simulink model "Flexible_Spacecraft"  (R2019a)
settings: Solver=ode4  StartTime=0.0  StopTime=10  FixedStep=0.005  RelTol=1e-3
libraries: aerolibconvert2 x5
settings Model: Creator=hoomaan  LastModifiedBy=hoomaan
settings DataIOCC: ReturnWorkspaceOutputs=off
settings DebuggingCC: ArithmeticOperatorsInVariantConditions=warning
settings SFSimCC: SimUseLocalCustomCode=off
settings RTWCC: RTWUseLocalCustomCode=off
settings CodeAppCC: StateflowObjectComments=on

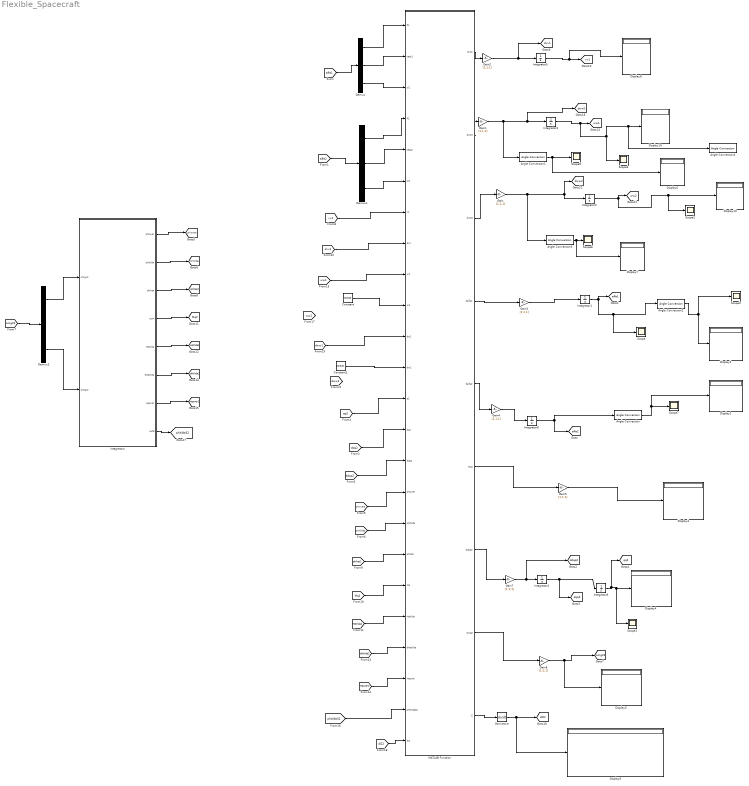
== system Flexible_Spacecraft ==
  Angle Conversion{,1..4} (5 alike) : aerolibconvert2/Angle Conversion  IU=rad  OU=deg
  Constant : Constant  Value=[0;0;0]
  Constant1 : Constant  Value=[0;0;0]
  Demux : Demux  Outputs=3
  Demux1 : Demux  Outputs=3
  Demux2 : Demux  Outputs=3
  Derivative : Derivative
  Display{1..10,13} (11 alike) : Display
  Gain{,1..5,7..8} (8 alike) : Gain  Gain=[1;1;1]
  Integrator{1..6,8} (7 alike) : Integrator  InitialCondition=[0;0;0]
  MATLAB Function : MATLAB Function  TreatAsAtomicUnit=on
  Scope{,1..7} (8 alike) : Scope
  integrators : MATLAB Function  TreatAsAtomicUnit=on
  tag scope: Hqover2=global, Hqtilda2=global, Mq2=global, alfa1=global, alfa2=global, dHtilda2=global, dI22=global, ddqq2=global, dqq2=global, dvv1=global, dww1=global, dww2=global, omg22=global, phihat2=global, phiover2=global, phitilda2=global, phitilda32=global, qq2=global, vv1=global, ww1=global, ww2=global
  wires:
  Angle Conversion/1 -> Scope7/1, Display1/1
  Integrator8/1 -> Angle Conversion/1, [alfa2]
  Integrator1/1 -> [alfa1], Scope/1, Angle Conversion2/1
  [alfa2] -> Demux1/1
  [alfa1] -> Demux/1
  Angle Conversion2/1 -> Scope3/1, Display2/1
  MATLAB Function/1(dv10) -> Gain2/1
  Integrator5/1 -> Display8/1, [vv1]
  MATLAB Function/2(dw10) -> Gain1/1
  MATLAB Function/3(dw20) -> Gain/1
  Integrator2/1 -> [ww2], Scope2/1, Display13/1
  [vv1] -> MATLAB Function/7(v1)
  [ww1] -> MATLAB Function/9(w1)
  [dww1] -> MATLAB Function/11(dw1)
  [dvv1] -> MATLAB Function/8(dv1)
  MATLAB Function/4(dalfa1) -> Gain3/1
  MATLAB Function/5(dalfa2) -> Gain4/1
  Gain/1 -> Angle Conversion3/1, Integrator2/1, [dww2]
  Gain1/1 -> Angle Conversion1/1, Integrator3/1, [dww1]
  Gain2/1 -> Integrator5/1, [dvv1]
  Gain3/1 -> Integrator1/1
  Gain4/1 -> Integrator8/1
  MATLAB Function/6(Mp2) -> Gain5/1
  Gain5/1 -> Display3/1
  Demux1/1 -> MATLAB Function/4(fi2)
  Demux1/2 -> MATLAB Function/5(teta2)
  Demux1/3 -> MATLAB Function/6(si2)
  Demux/1 -> MATLAB Function/1(fi1)
  Demux/2 -> MATLAB Function/2(teta1)
  Demux/3 -> MATLAB Function/3(si1)
  [dqq2] -> MATLAB Function/14(dq2)
  [ddqq2] -> MATLAB Function/15(ddq2)
  MATLAB Function/7(ddq20) -> Gain7/1
  Integrator4/1 -> [dqq2], Integrator6/1
  Integrator6/1 -> Scope1/1, Display4/1, [qq2]
  [qq2] -> MATLAB Function/13(q2)
  Gain7/1 -> [ddqq2], Integrator4/1
  MATLAB Function/8(omg2) -> Gain8/1
  Gain8/1 -> Display5/1, [omg22]
  [omg22] -> Demux2/1
  Demux2/1 -> integrators/1(omgx2)
  Demux2/3 -> integrators/2(omgz2)
  integrators/7(Hqover) -> [Hqover2]
  integrators/6(dHqtilda) -> [dHtilda2]
  integrators/5(Hqtilda) -> [Hqtilda2]
  integrators/4(out4) -> [Mq2]
  integrators/3(phihat) -> [phihat2]
  integrators/2(phitilda) -> [phitilda2]
  integrators/1(phiover) -> [phiover2]
  [phihat2] -> MATLAB Function/18(phihat)
  [phitilda2] -> MATLAB Function/17(phitilda)
  [phiover2] -> MATLAB Function/16(phiover)
  [Mq2] -> MATLAB Function/19(Mq)
  [Hqtilda2] -> MATLAB Function/20(Hqtilda)
  [dHtilda2] -> MATLAB Function/21(dHqtilda)
  [Hqover2] -> MATLAB Function/22(Hqover)
  Angle Conversion1/1 -> Display6/1, Scope5/1
  Angle Conversion3/1 -> Display7/1, Scope6/1
  integrators/8(out8) -> [phitilda32]
  [phitilda32] -> MATLAB Function/23(phitilda32)
  MATLAB Function/9(I2) -> Derivative/1
  Derivative/1 -> Display9/1, [dI22]
  [dI22] -> MATLAB Function/24(dI2)
  Constant/1 -> MATLAB Function/10(w2)
  Constant1/1 -> MATLAB Function/12(dw2)
  Integrator3/1 -> Scope4/1, Angle Conversion4/1, Display10/1, [ww1]

== matlab function Flexible_Spacecraft/integrators ==
  data: omgx2 input; phiover output; omgz2 input; phitilda output; phihat output; out4 output; Hqtilda output; dHqtilda output; Hqover output; out8 output
function [phiover,phitilda,phihat,out4,Hqtilda,dHqtilda,Hqover,out8] = integrators(omgx2,omgz2)
%#codegen

%    This function was generated by the Symbolic Math Toolbox version 7.1.
%    26-Feb-2017 23:02:28

phiover = reshape([0.0,0.0,0.0,0.0,-6.377876326171868,0.0,0.0,0.0,0.0],[3,3]);
if nargout > 1
    phitilda = reshape([0.0,0.0,0.0,0.0,0.0,-1.075141769112719e1,0.0,0.0,0.0],[3,3]);
end
if nargout > 2
    phihat = reshape([0.0,0.0,0.0,0.0,omgx2.*1.075141769112719e1,0.0,0.0,0.0,0.0],[3,3]);
end
if nargout > 3
    out4 = 1.008336895295853;
end
if nargout > 4
    t2 = reshape([0.0,0.0,0.0,0.0,0.0,0.0,0.0,0.0,0.0],[3,3]);
    Hqtilda = t2;
end
if nargout > 5
    dHqtilda = t2;
end
if nargout > 6
    Hqover = reshape([0.0,0.0,0.0,0.0,omgx2.^2.*(-1.008336895295853)-omgz2.^2.*1.008336895295853,0.0,0.0,0.0,0.0],[3,3]);
end
if nargout > 7
    out8 = -1.075141769112719e1;
end

== matlab function Flexible_Spacecraft/MATLAB Function ==
  data: fi1 input; teta1 input; dv10 output; dw10 output; dw20 output; si1 input; fi2 input; teta2 input; si2 input; v1 input; dv1 input; w1 input; w2 input; dw1 input; dw2 input; q2 input; dalfa1 output; dalfa2 output; Mp2 output; dq2 input; ddq20 output; ddq2 input; omg2 output; phiover input; phitilda input; phihat input; Mq input; Hqtilda input; dHqtilda input; Hqover input; phitilda32 input; dI2 input; I2 output
function [dv10,dw10,dw20,dalfa1,dalfa2,Mp2,ddq20,omg2,I2] = fcn(fi1,teta1,si1,fi2,teta2,si2,v1,dv1,w1,w2,dw1,dw2,q2,dq2,ddq2,phiover,phitilda,phihat,Mq,Hqtilda,dHqtilda,Hqover,phitilda32,dI2)

C10=[cos(teta1)*cos(si1) cos(fi1)*sin(si1)+sin(fi1)*sin(teta1)*cos(si1) sin(fi1)*sin(si1)-cos(fi1)*sin(teta1)*cos(si1);-cos(teta1)*sin(si1) cos(fi1)*cos(si1)-sin(fi1)*sin(teta1)*sin(si1) sin(fi1)*cos(si1)+cos(fi1)*sin(teta1)*sin(si1);sin(teta1) -sin(fi1)*cos(teta1) cos(fi1)*cos(teta1)];
C21=[1 0 0;0 1 0;0 0 1];
C12=C21';

D1=[cos(teta1)*cos(si1) sin(si1) 0;-cos(teta1)*sin(si1) cos(si1) 0;sin(teta1) 0 1];
D2=D1;

ro1=2740;
A1=1*1;
ro2=2740;
A2=1*0.01;
h2=0.01;

m1=2740;
m2=205.5;


r1=[1;0;0];
r2=[7.5;0;0];

s1=m1*[0.5;0;0];
s2=m2*[7.5/2;0;0];
j2=s2+(phiover*q2);

I1=[456.6666666667 0 0;0  1.141666666666667e+03 0;0 0  1.141666666666667e+03];
I2=[1.712671250000000e+01+(q2(2,1)*Mq*q2(2,1)) -phitilda32*q2(2,1) 0;-phitilda32*q2(2,1) 3.870250000000000e+03 0;0 0 3.853126712500000e+03+(q2(2,1)*Mq*q2(2,1))];
% dI2=[0 0 0;0 0 0;0 0 0];

k2=[0 0 0;0 34.0136 0;0 0 0];
c2=[0 0 0;0 2*0.01*sqrt(34.0136) 0;0 0 0];

M2=[0;0;0];
Q2=[0;0;0];
F1=[0;0;0];
M1=[20;100;125]+(C12*M2);



omg1=w1;

omg2=(C21*omg1)+w2;



v2=C21*(v1+((tilda(r1))'*omg1));



dC12=tilda(-(omg1)+(C12*omg2))*C12;
dC21=tilda(-(omg2)+(C21*omg1))*C21;

domg2=((dC21*w1)+(C21*dw1)+(dw2));

dv2=(dC21*v1)+(C21*dv1)+(dC21*(tilda(r1))'*w1)+(C21*(tilda(r1))'*dw1);



L1_v1=(m1*v1)+((tilda(s1))'*omg1);
L2_v2=(m2*v2)+((tilda(j2))'*omg2)+(phiover*dq2);
L1_omg1=(I1*omg1)+(tilda(s1)*v1);
L2_omg2=(I2*omg2)+(tilda(j2)*v2)+(phitilda*dq2);

Pv1=(L1_v1)+(C12*L2_v2);
Pw1=(L1_omg1)+(C12*tilda(r1)*L2_v2)+(C12*L2_omg2);
Pw2=L2_omg2;

dL1_v1=(m1*dv1)+((tilda(s1))'*dw1);
dL1_v1_hold=((tilda(s1))'*dw1);
dL2_v2=(m2*dv2)+((tilda(j2))'*domg2)+(tilda(omg2)*phiover*dq2)+(phiover*ddq2);
dL2_v2_hold=((tilda(j2))'*domg2)+(tilda(omg2)*phiover*dq2)+(phiover*ddq2);
dL1_omg1=(I1*dw1)+(tilda(s1)*dv1);
dL1_omg1_hold=(tilda(s1)*dv1);
dL2_omg2=(I2*domg2)+(dI2*omg2)+(tilda(s2)*dv2)-(tilda(v2)*phiover*dq2)+(phitilda*ddq2);
dL2_omg2_hold=(I2*C21*dw1)+(I2*dC21*w1)+(dI2*omg2)+(tilda(s2)*dv2)-(tilda(v2)*phiover*dq2)+(phitilda*ddq2);

dPv1=(dL1_v1_hold)+(C12*dL2_v2)+(dC12*L2_v2);

dPw1=(dL1_omg1_hold)+(dC12*tilda(r1)*L2_v2)+(C12*tilda(r1)*dL2_v2)+(dC12*L2_omg2)+(C12*dL2_omg2);

dPw2=dL2_omg2_hold;


Hold_dPv1=m1;
Hold_dPw1=I1;
Hold_dPw2=I2;

omg2_alfa2=-C21*tilda(w1)*C12;
v2_alfa2=-(C21*tilda(v1)*C12)-(C21*tilda((tilda(r1))'*omg1)*C12);

Mp2=(v2_alfa2*L2_v2)+(omg2_alfa2*L2_omg2);



dv10=(-dPv1-(tilda(w1)*Pv1)+F1)/(Hold_dPv1);
dw10=inv(Hold_dPw1)*(-dPw1-(tilda(v1)*Pv1)-(tilda(w1)*Pw1)+M1);
dw20=inv(Hold_dPw2)*(-dPw2-(tilda(w2)*Pw2)+Mp2+M2);
ddq20=-inv(Mq)*((phiover'*dv2)+(phitilda'*domg2)+(dHqtilda*q2)+(Hqtilda*dq2)+(Hqover*q2)-(phihat'*omg2)+(phiover'*tilda(omg2)*v2)+(Hqtilda*dq2)+(k2*q2)+(c2*dq2)-(Q2));



dalfa1=inv(D1)*[w1(1,1);w1(2,1);w1(3,1)];
dalfa2=inv(D2)*[w2(1,1);w2(2,1);w2(3,1)];
